simulink model "lotka_voltera_dx1"  (Simulink 7.8)
settings: Solver=ode4  StartTime=0.0  StopTime=time_span  RelTol=1e-3
values from neighbouring files (symbols this model uses):
  IC = [x_i(i),y_i(j)]    [run_lotka_voltera.m]
  samp_time = .025    (= 0.025)    [run_ODE6.m]    (also in run_lotka_voltera.m)
undefined symbols (not defined in the file or in its folder): c4, c5, c6, outstr
settings Model: Creator=Kourosh Danai  LastModifiedBy=BionicBill
settings DataIOCC: SaveFormat=StructureWithTime  TimeSaveName=t  OutputSaveName=y
settings DebuggingCC: AlgebraicLoopMsg=none  FcnCallInpInsideContextMsg=Use local settings  StrictBusMsg=Warning
settings SFSimCC: SimParseCustomCode=off

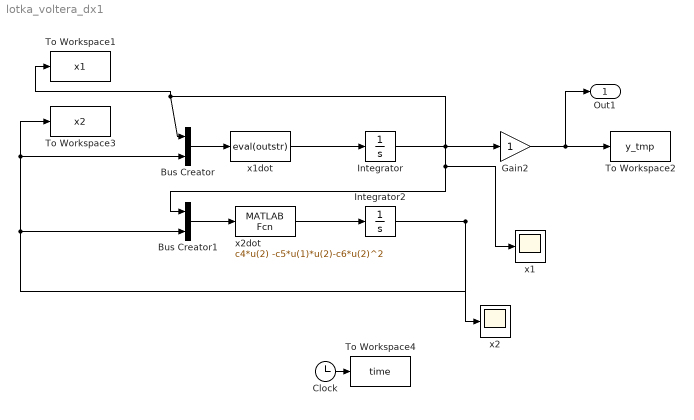
== system lotka_voltera_dx1 ==
  Bus Creator : BusCreator  Inputs=2
  Bus Creator1 : BusCreator  Inputs=2
  Clock : Clock
  Gain2 : Gain
  Integrator : Integrator  InitialCondition=IC(1)
  Integrator2 : Integrator  InitialCondition=IC(2)
  To Workspace1 : ToWorkspace  VariableName=x1  SampleTime=-1  SaveFormat=Structure
  To Workspace2 : ToWorkspace  VariableName=y_tmp  SampleTime=-1  SaveFormat=Array
  To Workspace3 : ToWorkspace  VariableName=x2  SampleTime=-1  SaveFormat=Structure
  To Workspace4 : ToWorkspace  VariableName=time  SampleTime=-1  SaveFormat=Array
  x1 : Scope
  x1dot : MATLABFcn  MATLABFcn=eval(outstr)  SampleTime=samp_time
  x2 : Scope
      settings: SaveName=ScopeData2
  x2dot : MATLABFcn  MATLABFcn=c4*u(2) -c5*u(1)*u(2)-c6*u(2)^2
  Out1 : Outport
  wires:
  Bus Creator/1 -> x1dot/1
  Bus Creator1/1 -> x2dot/1
  Integrator/1 -> Bus Creator1/1, x1/1, Bus Creator/1, To Workspace1/1, Gain2/1
  Integrator2/1 -> x2/1, Bus Creator/2, To Workspace3/1, Bus Creator1/2
  Gain2/1 -> To Workspace2/1, Out1/1
  x1dot/1 -> Integrator/1
  x2dot/1 -> Integrator2/1
  Clock/1 -> To Workspace4/1
